simulink model "buck_boost_ZN"  (R2025a)
settings: Solver=FixedStepAuto  StartTime=0.0  StopTime=15  FixedStep=0.001  RelTol=1e-3
values from neighbouring files (symbols this model uses):
  C = 470e-6    (= 0.00047)    [projekat_1.m]
  E = 12    [projekat_1.m]
  L = 15.91e-3    (= 0.01591)    [projekat_1.m]
  noise_var = (0.03*x2_eq)^2    (= 0.455625)    [projekat_1.m]
  R = 52    [projekat_1.m]
  u_eq = eval(u_eq)    [projekat_1.m]
  x2_eq = -22.5    [projekat_1.m]
settings Model: Creator=PC  LastModifiedBy=PC
settings DataIOCC: ReturnWorkspaceOutputs=off

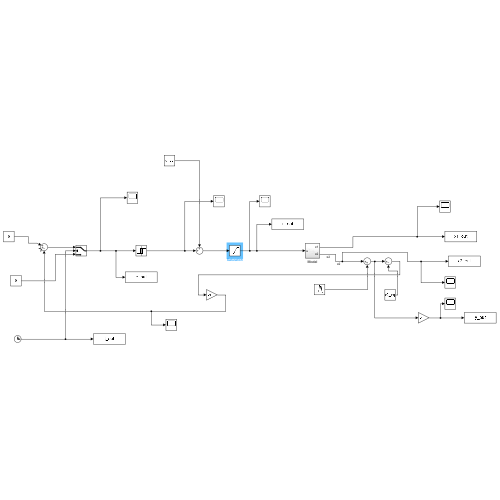
[thumbnail: Simulink's stored preview of the top-level diagram]
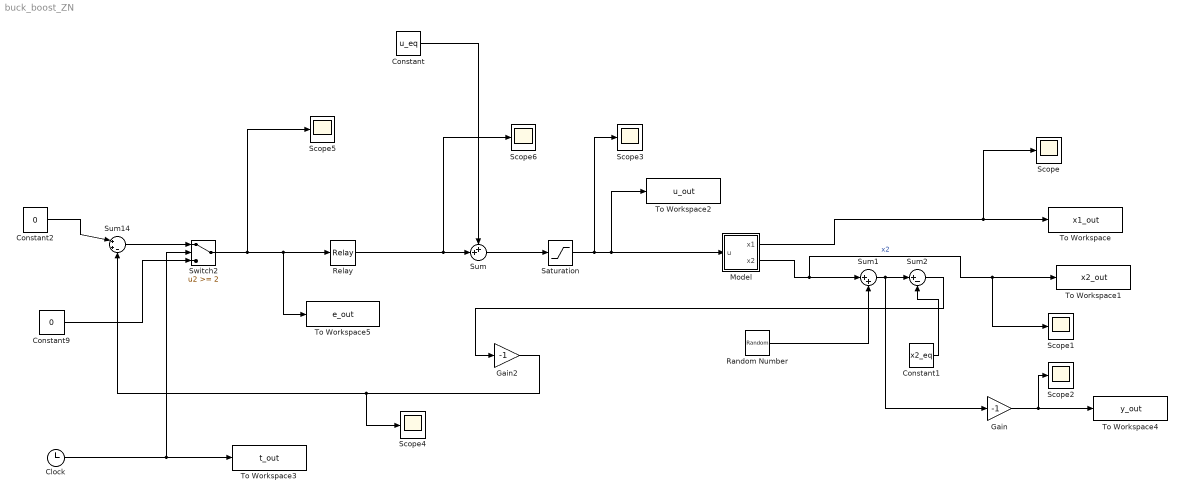
== system buck_boost_ZN ==
  Clock : Clock
  Constant : Constant  Value=u_eq
  Constant1 : Constant  Value=x2_eq
  Constant2 : Constant  Value=0
  Constant9 : Constant  Value=0
  Gain : Gain  Gain=-1
  Gain2 : Gain  Gain=-1
  Model : Subsystem
  Random Number : RandomNumber  Variance=noise_var  SampleTime=0.001
  Relay : Relay  OnSwitchValue=0  OffSwitchValue=0  OnOutputValue=u_eq*0.1  OffOutputValue=-u_eq*0.1
  Saturation : Saturate  UpperLimit=0.90  LowerLimit=0.20
  Scope{,1..6} (7 alike) : Scope
      Scope settings: ActiveDisplayYMinimum=-1  ActiveDisplayYMaximum=1
      Scope1 settings: ActiveDisplayYMinimum=-17.390570872112225  ActiveDisplayYMaximum=17.699619428483988
      Scope2 settings: ActiveDisplayYMinimum=-1.226762900906336E+223  ActiveDisplayYMaximum=1.0997258244058199E+223  DataLoggingVariableName=ScopeData2
      Scope3 settings: ActiveDisplayYMinimum=0.32966598731056374  ActiveDisplayYMaximum=1.018752292305293  DataLoggingVariableName=ScopeData3
      Scope4 settings: ActiveDisplayYMinimum=-20.327822254462426  ActiveDisplayYMaximum=5.8570180187516909  DataLoggingVariableName=ScopeData4
      Scope5 settings: ActiveDisplayYMinimum=-0.83588221436992782  ActiveDisplayYMaximum=30.064451899251992  DataLoggingVariableName=ScopeData5
      Scope6 settings: ActiveDisplayYMinimum=-132.7226298777324  ActiveDisplayYMaximum=31.716936684348454  DataLoggingVariableName=ScopeData6
  Sum : Sum  Inputs=++|
  Sum1 : Sum  Inputs=|++
  Sum14 : Sum  Inputs=|++-
  Sum2 : Sum  Inputs=|+-
  Switch2 : Switch  Threshold=2  SaturateOnIntegerOverflow=off  InputSameDT=off
  To Workspace : ToWorkspace  VariableName=x1_out  SampleTime=-1
  To Workspace1 : ToWorkspace  VariableName=x2_out  SampleTime=-1
  To Workspace2 : ToWorkspace  VariableName=u_out  SampleTime=-1
  To Workspace3 : ToWorkspace  VariableName=t_out  SampleTime=-1
  To Workspace4 : ToWorkspace  VariableName=y_out  SampleTime=-1
  To Workspace5 : ToWorkspace  VariableName=e_out  SampleTime=-1
  wires:
  Saturation/1 -> Scope3/1, To Workspace2/1, Model/1(u)
  Model/1(x1) -> Scope/1, To Workspace/1
  Gain/1 -> To Workspace4/1, Scope2/1
  Random Number/1 -> Sum1/2
  Sum/1 -> Saturation/1
  Constant/1 -> Sum/1
  Constant9/1 -> Switch2/3
  Sum14/1 -> Switch2/1
  Constant2/1 -> Sum14/1
  Model/2(x2) -> Sum1/1, Scope1/1, To Workspace1/1  "x2"
  Constant1/1 -> Sum2/2
  Clock/1 -> Switch2/2, To Workspace3/1
  Gain2/1 -> Scope4/1, Sum14/3
  Sum1/1 -> Gain/1, Sum2/1
  Sum2/1 -> Gain2/1
  Relay/1 -> Scope6/1, Sum/2
  Switch2/1 -> To Workspace5/1, Relay/1, Scope5/1

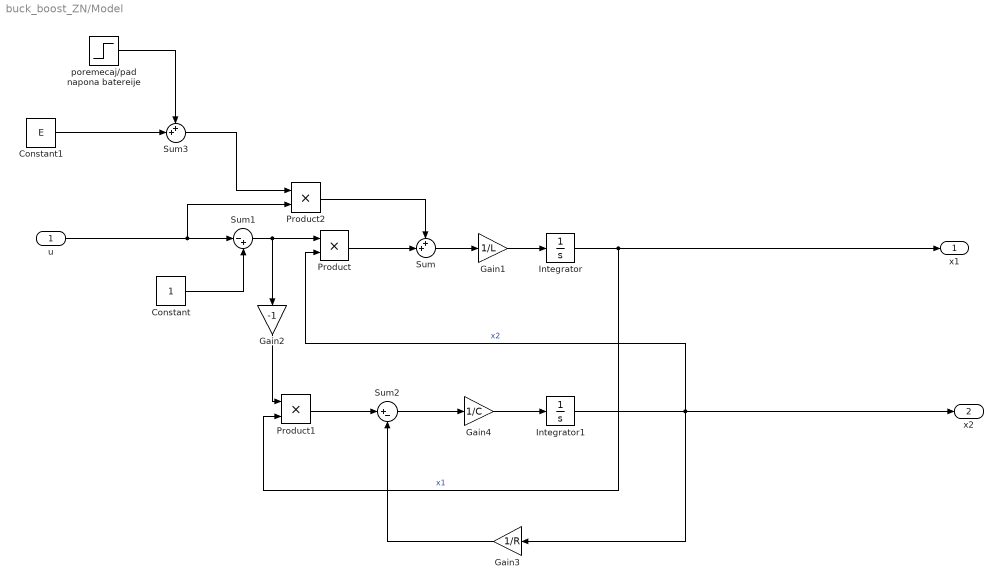
== system buck_boost_ZN/Model ==
  u : Inport
  Constant : Constant
  Constant1 : Constant  Value=E
  Gain1 : Gain  Gain=1/L
  Gain2 : Gain  Gain=-1
  Gain3 : Gain  Gain=1/R
  Gain4 : Gain  Gain=1/C
  Integrator : Integrator
  Integrator1 : Integrator
  Product : Product
  Product1 : Product
  Product2 : Product
  Sum : Sum  Inputs=++|
  Sum1 : Sum  Inputs=|-+
  Sum2 : Sum  Inputs=|+-
  Sum3 : Sum  Inputs=++|
  poremecaj/pad napona batereije : Step  Time=10  After=-1  SampleTime=0
  x1 : Outport
  x2 : Outport  Port=2
  wires:
  Product1/1 -> Sum2/1
  Integrator1/1 -> x2/1, Gain3/1, Product/2  "x2"
  Gain3/1 -> Sum2/2
  Constant/1 -> Sum1/2
  Sum2/1 -> Gain4/1
  Product/1 -> Sum/2
  Gain1/1 -> Integrator/1
  Sum1/1 -> Product/1, Gain2/1
  Integrator/1 -> x1/1, Product1/2  "x1"
  Product2/1 -> Sum/1
  u/1 -> Product2/2, Sum1/1
  Gain4/1 -> Integrator1/1
  Sum/1 -> Gain1/1
  Gain2/1 -> Product1/1
  Constant1/1 -> Sum3/2
  poremecaj/pad napona batereije/1 -> Sum3/1
  Sum3/1 -> Product2/1
